simulink model "nominal_drift_REALTIME"  (R2020b)
settings: Solver=FixedStepDiscrete  StartTime=0.0  StopTime=10.0  RelTol=1e-3  EnableMultiTasking=on
values from neighbouring files (symbols this model uses):
  denHw = [0.03 0 0 0]    [data_v2_500.mat]    (also in data_v6_nominaldrift500.mat)
  denLPFz = [1 -0.978482055734]    [data_v2_500.mat]    (also in data_v6_nominaldrift500.mat)
  drv =     [data_v2_500.mat]    (also in data_v6_nominaldrift500.mat)
  gbox =     [data_v2_500.mat]    (also in data_v6_nominaldrift500.mat)
  N_u = 0    [data_v2_500.mat]    (also in data_v6_nominaldrift500.mat)
  N_x = [1 0 0 0]    [data_v2_500.mat]    (also in data_v6_nominaldrift500.mat)
  numHw = [1 0 0 -1]    [data_v2_500.mat]    (also in data_v6_nominaldrift500.mat)
  numLPFz = [0.0215179442657 0]    [data_v2_500.mat]    (also in data_v6_nominaldrift500.mat)
  sens =     [data_v2_500.mat]    (also in data_v6_nominaldrift500.mat)
  Ts = 0.01    [data_v2_500.mat]    (also in data_v6_nominaldrift500.mat)
  wheel =     [data_v2_500.mat]    (also in data_v6_nominaldrift500.mat)
undefined symbols (not defined in the file or in its folder): C_gain, DiscIntNeverNeededParam, T
libraries: BalRobTbx_baselib x9
settings Model: SILPILModeSetting=veronly  ExtModeTrigDuration=2  Creator=39345  LastModifiedBy=pavarinlau
settings DataIOCC: ReturnWorkspaceOutputs=off
settings OptimizationCC: EnhancedBackFolding=on  PassReuseOutputArgsAs=Individual arguments  ZeroExternalMemoryAtStartup=off  ZeroInternalMemoryAtStartup=off  MaxStackSize=64  OptimizeBlockOrder=speed  DifferentSizesBufferReuse=on  OptimizationCustomize=off  EfficientTunableParamExpr=on
settings DebuggingCC: ParameterTunabilityLossMsg=error
settings HardwareCC: ProdBitPerInt=16  ProdBitPerPointer=16  ProdBitPerSizeT=16  ProdBitPerPtrDiffT=16  ProdLargestAtomicFloat=None  ProdWordSize=8  ProdHWDeviceType=Atmel->AVR
settings SFSimCC: MATLABDynamicMemAlloc=off
settings RTWCC: Description=Embedded Coder  SystemTargetFile=ert.tlc  HardwareBoard=Arduino Mega 2560  TemplateMakefile=ert_default_tmf  GenerateReport=on  Toolchain=Arduino AVR  BuildConfiguration=Faster Runs
settings CodeAppCC: ForceParamTrailComments=on  IgnoreCustomStorageClasses=off  OperatorAnnotations=on  SimulinkDataObjDesc=on  SFDataObjDesc=on  InsertBlockDesc=on
settings ERTTargetCC: SupportContinuousTime=on  SupportVariableSizeSignals=on  ExtModeStaticAllocSize=2048

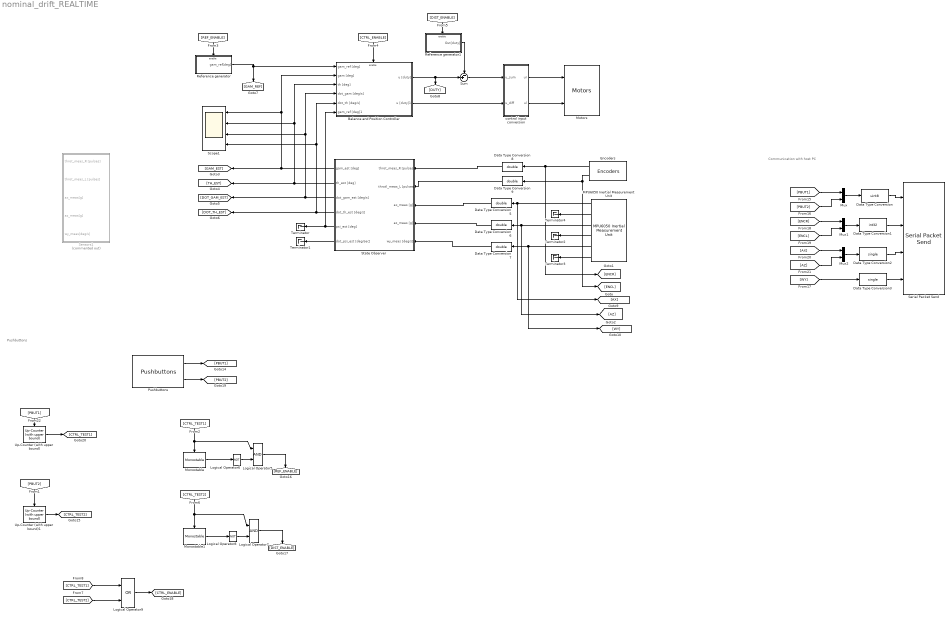
== system nominal_drift_REALTIME ==
  note: Communication with host PC
  note: Pushbuttons
  Balance and Position Controller : Subsystem
  Data Type Conversion : DataTypeConversion  OutDataTypeStr=uint8
  Data Type Conversion1 : DataTypeConversion  OutDataTypeStr=int32
  Data Type Conversion2 : DataTypeConversion  OutDataTypeStr=single
  Data Type Conversion3 : DataTypeConversion  OutDataTypeStr=single
  Data Type Conversion{5..9} (5 alike) : DataTypeConversion  OutDataTypeStr=double
  Encoders : BalRobTbx_baselib/Inputs/Encoders
      settings: SourceProductName=Balancing Robot Toolbox
  Logical Operator5 : Logic  AllPortsSameDT=off  OutDataTypeStr=boolean
  Logical Operator6 : Logic  Operator=NOT  Inputs=1  AllPortsSameDT=off  OutDataTypeStr=boolean
  Logical Operator7 : Logic  AllPortsSameDT=off  OutDataTypeStr=boolean
  Logical Operator8 : Logic  Operator=NOT  Inputs=1  AllPortsSameDT=off  OutDataTypeStr=boolean
  Logical Operator9 : Logic  Operator=OR  AllPortsSameDT=off  OutDataTypeStr=boolean
  MPU6050 Inertial Measurement Unit : BalRobTbx_baselib/Inputs/MPU6050 Inertial Measurement Unit
      settings: SourceProductName=Balancing Robot Toolbox
  Monostable : BalRobTbx_baselib/Utilities/Monostable  Tp=10
      settings: SourceProductName=Balancing Robot Toolbox
  Monostable1 : BalRobTbx_baselib/Utilities/Monostable  Tp=10
      settings: SourceProductName=Balancing Robot Toolbox
  Motors : BalRobTbx_baselib/Outputs/Motors
      settings: SourceProductName=Balancing Robot Toolbox
  Mux : Mux  Inputs=2
  Mux1 : Mux  Inputs=2
  Mux2 : Mux  Inputs=2
  Pushbuttons : BalRobTbx_baselib/Inputs/Pushbuttons
      settings: SourceProductName=Balancing Robot Toolbox
  Reference generator : Subsystem
  Reference generator1 : Subsystem
  Scope1 : Scope  NumInputPorts=4
  Sensors1 : Subsystem  Commented=on
  Serial Packet Send : BalRobTbx_baselib/Communication/Serial Packet Send  serialLinkOpt=Bluetooth  baudRateOpt=38400  waitHostTxCmd=on  txStartCmd=65  txStopCmd=66  packetSpec={'2*uint8', '2*int32', '2*single', 'single'}  cobsEncoded=on  nullTerminated=on  showEnablePort=off
      settings: SourceProductName=Balancing Robot Toolbox
  State Observer : Subsystem
  Sum : Sum  Inputs=-+|
  Terminator{,1..4} (5 alike) : Terminator
  Up-Counter (with upper bound) : BalRobTbx_baselib/Utilities/Up-Counter (with upper bound)  CMAX=10  C0=0
      settings: SourceProductName=Balancing Robot Toolbox
  Up-Counter (with upper bound)1 : BalRobTbx_baselib/Utilities/Up-Counter (with upper bound)  CMAX=10  C0=0
      settings: SourceProductName=Balancing Robot Toolbox
  control input conversion : Subsystem
  wires:
  Balance and Position Controller/2(u [duty]1) -> control input conversion/2(u_diff)
  State Observer/5(psi_est [deg]) -> Terminator/1, Balance and Position Controller/6(gam_ref [deg]1)
  [REF_ENABLE] -> Reference generator/Enable
  State Observer/1(gam_est [deg]) -> Balance and Position Controller/2(gam [deg]), Scope1/1, [GAM_EST]
  State Observer/2(th_est [deg]) -> Balance and Position Controller/3(th [deg]), Scope1/2, [TH_EST]
  Data Type Conversion6/1 -> State Observer/4("az_meas [g] ")
  Reference generator/1(gam_ref[deg]) -> Balance and Position Controller/1(gam_ref [deg]), [GAM_REF]
  [CTRL_ENABLE] -> Balance and Position Controller/Enable
  Sum/1 -> control input conversion/1(u_sum)
  Data Type Conversion9/1 -> State Observer/2(throtl_meas_L [pulses])
  State Observer/4(dot_th_est [deg/s]) -> Balance and Position Controller/5(dot_th [deg/s]), Scope1/4, [DOT_TH_EST]
  Reference generator1/1(Out[duty]) -> Sum/1
  State Observer/6(dot_psi_est [deg/sec]) -> Terminator1/1
  Data Type Conversion8/1 -> State Observer/1("throt_meas_R [pulses] ")
  State Observer/3(dot_gam_est [deg/s]) -> Balance and Position Controller/4(dot_gam [deg/s]), Scope1/3, [DOT_GAM_EST]
  Data Type Conversion7/1 -> State Observer/5(wy_meas [deg/s])
  [DIST_ENABLE] -> Reference generator1/Enable
  Balance and Position Controller/1(u [duty]) -> [DUTY], Sum/2
  Data Type Conversion3/1 -> Serial Packet Send/4
  Mux2/1 -> Data Type Conversion2/1
  Data Type Conversion2/1 -> Serial Packet Send/3
  [WY] -> Data Type Conversion3/1
  Data Type Conversion1/1 -> Serial Packet Send/2
  [ENCR] -> Mux1/1
  [PBUT2] -> Mux/2
  [PBUT1] -> Mux/1
  Mux/1 -> Data Type Conversion/1
  [AX] -> Mux2/1
  [ENCL] -> Mux1/2
  [AZ] -> Mux2/2
  Data Type Conversion/1 -> Serial Packet Send/1
  Mux1/1 -> Data Type Conversion1/1
  [PBUT1] -> Up-Counter (with upper bound)/Trigger
  Up-Counter (with upper bound)/1 -> [CTRL_TEST1]
  Up-Counter (with upper bound)1/1 -> [CTRL_TEST2]
  Monostable/1 -> Logical Operator6/1
  Pushbuttons/2 -> [PBUT2]
  Logical Operator7/1 -> [DIST_ENABLE]
  Pushbuttons/1 -> [PBUT1]
  [CTRL_TEST2] -> Logical Operator9/2
  Logical Operator6/1 -> Logical Operator5/2
  [CTRL_TEST2] -> Logical Operator7/1, Monostable1/Enable
  Logical Operator9/1 -> [CTRL_ENABLE]
  [PBUT2] -> Up-Counter (with upper bound)1/Trigger
  [CTRL_TEST1] -> Monostable/Enable, Logical Operator5/1
  [CTRL_TEST1] -> Logical Operator9/1
  Logical Operator5/1 -> [REF_ENABLE]
  Monostable1/1 -> Logical Operator8/1
  Logical Operator8/1 -> Logical Operator7/2
  Encoders/1 -> [ENCR], Data Type Conversion8/1
  MPU6050 Inertial Measurement Unit/5 -> [WY], Data Type Conversion7/1
  MPU6050 Inertial Measurement Unit/2 -> Terminator4/1
  MPU6050 Inertial Measurement Unit/3 -> [AZ], Data Type Conversion6/1
  MPU6050 Inertial Measurement Unit/6 -> Terminator3/1
  MPU6050 Inertial Measurement Unit/1 -> [AX], Data Type Conversion5/1
  MPU6050 Inertial Measurement Unit/4 -> Terminator2/1
  Encoders/2 -> [ENCL], Data Type Conversion9/1
  Data Type Conversion5/1 -> State Observer/3("ax_meas [g] ")
  control input conversion/1(ur) -> Motors/1
  control input conversion/2(ul) -> Motors/2

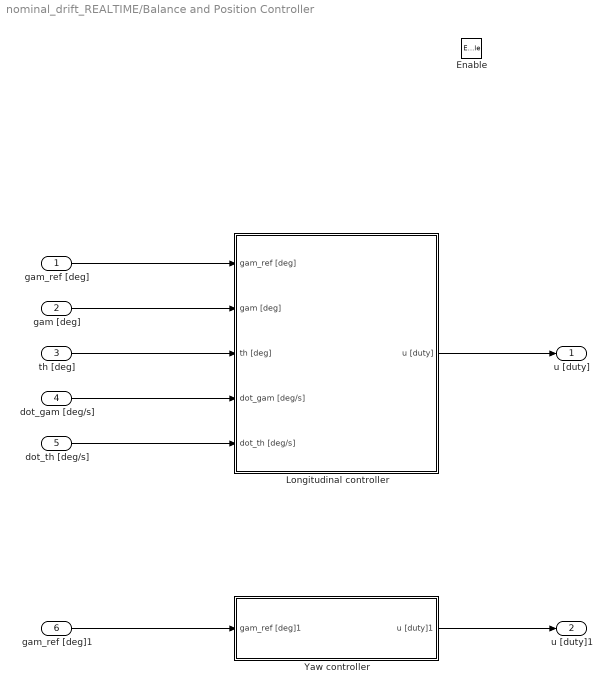
== system nominal_drift_REALTIME/Balance and Position Controller ==
  gam_ref [deg] : Inport
  gam [deg] : Inport  Port=2
  th [deg] : Inport  Port=3
  dot_gam [deg/s] : Inport  Port=4
  dot_th [deg/s] : Inport  Port=5
  gam_ref [deg]1 : Inport  Port=6
  Enable : EnablePort  StatesWhenEnabling=reset
  Longitudinal controller : Subsystem
  Yaw controller : Subsystem
  u [duty] : Outport
  u [duty]1 : Outport  Port=2  InitialOutput=[0]
  wires:
  gam_ref [deg]/1 -> Longitudinal controller/1(gam_ref [deg])
  Longitudinal controller/1(u [duty]) -> u [duty]/1
  gam [deg]/1 -> Longitudinal controller/2(gam [deg])
  th [deg]/1 -> Longitudinal controller/3(th [deg])
  dot_th [deg/s]/1 -> Longitudinal controller/5(dot_th [deg/s])
  dot_gam [deg/s]/1 -> Longitudinal controller/4(dot_gam [deg/s])
  Yaw controller/1(u [duty]1) -> u [duty]1/1
  gam_ref [deg]1/1 -> Yaw controller/1(gam_ref [deg]1)

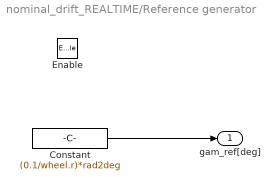
== system nominal_drift_REALTIME/Reference generator ==
  Enable : EnablePort  StatesWhenEnabling=reset
  Constant : Constant  Value=(0.1/wheel.r)*rad2deg  SampleTime=0.01
  gam_ref[deg] : Outport
  wires:
  Constant/1 -> gam_ref[deg]/1

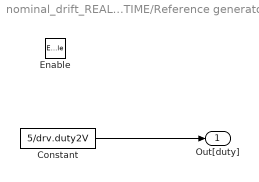
== system nominal_drift_REALTIME/Reference generator1 ==
  Enable : EnablePort  StatesWhenEnabling=reset
  Constant : Constant  Value=5/drv.duty2V  SampleTime=0.01
  Out[duty] : Outport  InitialOutput=[0]
  wires:
  Constant/1 -> Out[duty]/1

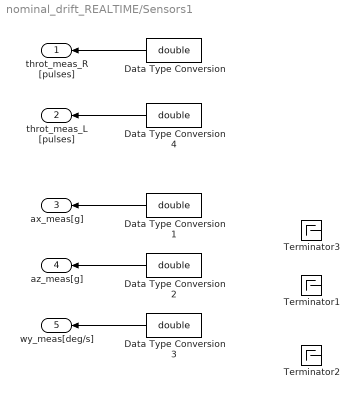
== system nominal_drift_REALTIME/Sensors1 ==
  Data Type Conversion{,1..4} (5 alike) : DataTypeConversion  OutDataTypeStr=double
  Terminator1 : Terminator
  Terminator2 : Terminator
  Terminator3 : Terminator
  throt_meas_R [pulses] : Outport
  throt_meas_L [pulses] : Outport  Port=2
  ax_meas[g] : Outport  Port=3
  az_meas[g] : Outport  Port=4
  wy_meas[deg/s] : Outport  Port=5
  wires:
  Data Type Conversion/1 -> throt_meas_R [pulses]/1
  Data Type Conversion1/1 -> ax_meas[g]/1
  Data Type Conversion2/1 -> az_meas[g]/1
  Data Type Conversion3/1 -> wy_meas[deg/s]/1
  Data Type Conversion4/1 -> throt_meas_L [pulses]/1

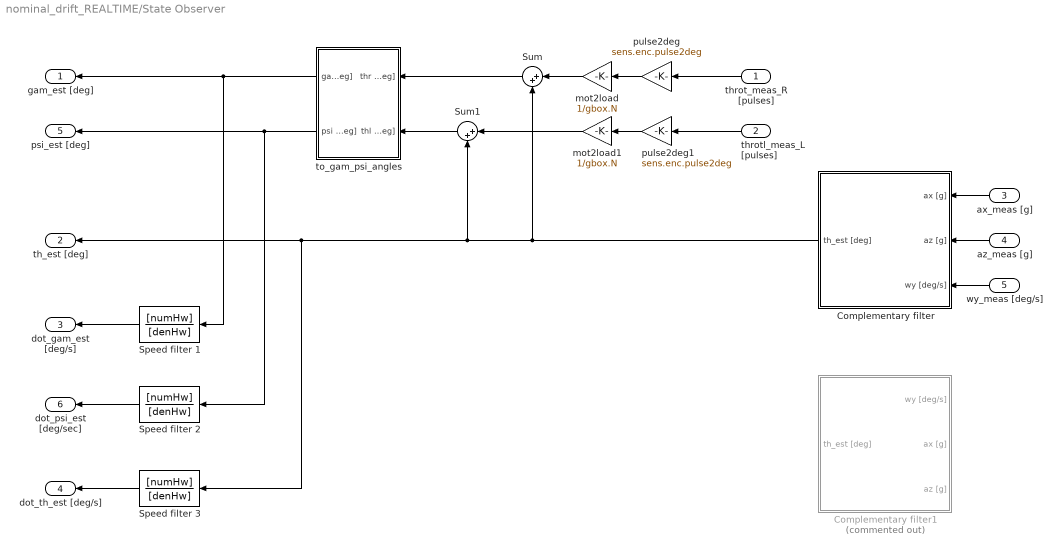
== system nominal_drift_REALTIME/State Observer ==
  "throt_meas_R [pulses] " : Inport
  throtl_meas_L [pulses] : Inport  Port=2
  "ax_meas [g] " : Inport  Port=3
  "az_meas [g] " : Inport  Port=4
  wy_meas [deg/s] : Inport  Port=5
  Complementary filter : Subsystem
  Complementary filter1 : Subsystem  Commented=on
  Speed filter 1 : DiscreteTransferFcn  Numerator=[numHw]  Denominator=[denHw]  SampleTime=Ts
  Speed filter 2 : DiscreteTransferFcn  Numerator=[numHw]  Denominator=[denHw]  SampleTime=Ts
  Speed filter 3 : DiscreteTransferFcn  Numerator=[numHw]  Denominator=[denHw]  SampleTime=Ts
  Sum : Sum  Inputs=|++
  Sum1 : Sum  Inputs=|++
  mot2load : Gain  Gain=1/gbox.N
  mot2load1 : Gain  Gain=1/gbox.N
  pulse2deg : Gain  Gain=sens.enc.pulse2deg
  pulse2deg1 : Gain  Gain=sens.enc.pulse2deg
  to_gam_psi_angles : Subsystem
  gam_est [deg] : Outport
  th_est [deg] : Outport  Port=2
  dot_gam_est [deg/s] : Outport  Port=3
  dot_th_est [deg/s] : Outport  Port=4
  psi_est [deg] : Outport  Port=5
  dot_psi_est [deg/sec] : Outport  Port=6
  wires:
  pulse2deg/1 -> mot2load/1
  "throt_meas_R [pulses] "/1 -> pulse2deg/1
  mot2load/1 -> Sum/1
  Complementary filter/1("th_est [deg] ") -> Sum/2, th_est [deg]/1, Speed filter 3/1, Sum1/2
  Speed filter 1/1 -> dot_gam_est [deg/s]/1
  Speed filter 3/1 -> dot_th_est [deg/s]/1
  "ax_meas [g] "/1 -> Complementary filter/1("ax [g] ")
  "az_meas [g] "/1 -> Complementary filter/2("az [g] ")
  wy_meas [deg/s]/1 -> Complementary filter/3(wy [deg/s])
  throtl_meas_L [pulses]/1 -> pulse2deg1/1
  pulse2deg1/1 -> mot2load1/1
  mot2load1/1 -> Sum1/1
  Sum1/1 -> to_gam_psi_angles/2(thl [deg])
  Sum/1 -> to_gam_psi_angles/1(thr [deg])
  to_gam_psi_angles/1(gam [deg]) -> Speed filter 1/1, gam_est [deg]/1
  to_gam_psi_angles/2(psi [deg]) -> Speed filter 2/1, psi_est [deg]/1
  Speed filter 2/1 -> dot_psi_est [deg/sec]/1

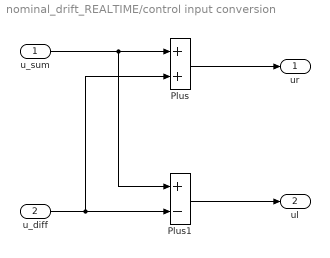
== system nominal_drift_REALTIME/control input conversion ==
  u_sum : Inport
  u_diff : Inport  Port=2
  Plus : Sum
  Plus1 : Sum  Inputs=+-
  ur : Outport
  ul : Outport  Port=2
  wires:
  u_sum/1 -> Plus1/1, Plus/1
  u_diff/1 -> Plus1/2, Plus/2
  Plus/1 -> ur/1
  Plus1/1 -> ul/1

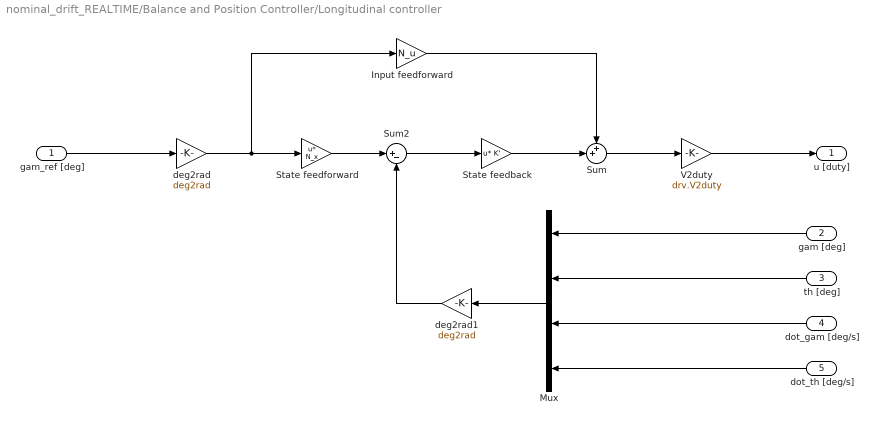
== system nominal_drift_REALTIME/Balance and Position Controller/Longitudinal controller ==
  gam_ref [deg] : Inport
  gam [deg] : Inport  Port=2
  th [deg] : Inport  Port=3
  dot_gam [deg/s] : Inport  Port=4
  dot_th [deg/s] : Inport  Port=5
  Input feedforward : Gain  Gain=N_u
  Mux : Mux
  State feedback : Gain  Gain=K'  Multiplication=Matrix(u*K)
  "State feedforward\t" : Gain  Gain=N_x  Multiplication=Matrix(u*K)
  Sum : Sum  Inputs=++|
  Sum2 : Sum  Inputs=|+-
  V2duty : Gain  Gain=drv.V2duty
  deg2rad : Gain  Gain=deg2rad
  deg2rad1 : Gain  Gain=deg2rad
  u [duty] : Outport
  wires:
  Mux/1 -> deg2rad1/1
  Sum2/1 -> State feedback/1
  deg2rad/1 -> Input feedforward/1, "State feedforward\t"/1
  dot_gam [deg/s]/1 -> Mux/3
  State feedback/1 -> Sum/2
  "State feedforward\t"/1 -> Sum2/1
  deg2rad1/1 -> Sum2/2
  Sum/1 -> V2duty/1
  dot_th [deg/s]/1 -> Mux/4
  Input feedforward/1 -> Sum/1
  gam_ref [deg]/1 -> deg2rad/1
  gam [deg]/1 -> Mux/1
  th [deg]/1 -> Mux/2
  V2duty/1 -> u [duty]/1

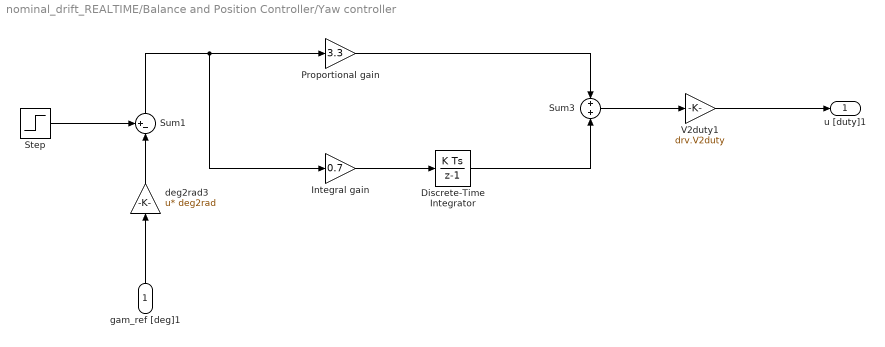
== system nominal_drift_REALTIME/Balance and Position Controller/Yaw controller ==
  gam_ref [deg]1 : Inport
  Discrete-Time Integrator : DiscreteIntegrator  SampleTime=-1  ICPrevOutput=DiscIntNeverNeededParam  ICPrevScaledInput=DiscIntNeverNeededParam
  Integral gain : Gain  Gain=0.7
  Proportional gain : Gain  Gain=3.3
  Step : Step  Time=0  After=0  SampleTime=0
  Sum1 : Sum  Inputs=+-|
  Sum3 : Sum  Inputs=+|+
  V2duty1 : Gain  Gain=drv.V2duty
  deg2rad3 : Gain  Gain=deg2rad  Multiplication=Matrix(u*K)
  u [duty]1 : Outport
  wires:
  gam_ref [deg]1/1 -> deg2rad3/1
  Sum1/1 -> Integral gain/1, Proportional gain/1
  Step/1 -> Sum1/1
  Integral gain/1 -> Discrete-Time Integrator/1
  deg2rad3/1 -> Sum1/2
  V2duty1/1 -> u [duty]1/1
  Proportional gain/1 -> Sum3/1
  Discrete-Time Integrator/1 -> Sum3/2
  Sum3/1 -> V2duty1/1

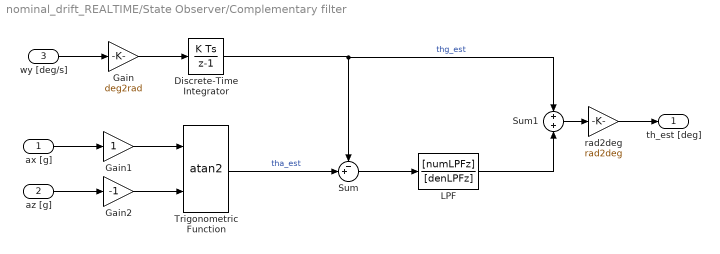
== system nominal_drift_REALTIME/State Observer/Complementary filter ==
  "ax [g] " : Inport
  "az [g] " : Inport  Port=2
  wy [deg/s] : Inport  Port=3
  Discrete-Time Integrator : DiscreteIntegrator  gainval=1  SampleTime=Ts  ICPrevOutput=DiscIntNeverNeededParam  ICPrevScaledInput=DiscIntNeverNeededParam
  Gain : Gain  Gain=deg2rad
  Gain1 : Gain
  Gain2 : Gain  Gain=-1
  LPF : DiscreteTransferFcn  Numerator=[numLPFz]  Denominator=[denLPFz]  SampleTime=Ts
  Sum : Sum  Inputs=-+|
  Sum1 : Sum
  Trigonometric Function : Trigonometry  Operator=atan2
  rad2deg : Gain  Gain=rad2deg
  "th_est [deg] " : Outport
  wires:
  "az [g] "/1 -> Gain2/1
  "ax [g] "/1 -> Gain1/1
  wy [deg/s]/1 -> Gain/1
  Gain/1 -> Discrete-Time Integrator/1
  Gain2/1 -> Trigonometric Function/2
  Gain1/1 -> Trigonometric Function/1
  Trigonometric Function/1 -> Sum/2  "tha_est"
  Discrete-Time Integrator/1 -> Sum1/1, Sum/1  "thg_est"
  rad2deg/1 -> "th_est [deg] "/1
  Sum1/1 -> rad2deg/1
  Sum/1 -> LPF/1
  LPF/1 -> Sum1/2

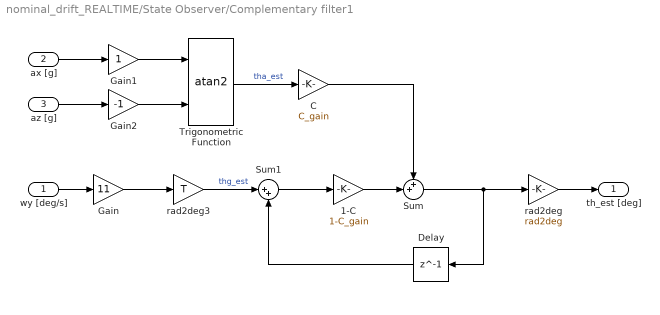
== system nominal_drift_REALTIME/State Observer/Complementary filter1 ==
  wy [deg/s] : Inport
  "ax [g] " : Inport  Port=2
  "az [g] " : Inport  Port=3
  1-C : Gain  Gain=1-C_gain
  C : Gain  Gain=C_gain
  Delay : Delay  DelayLength=1
  Gain : Gain  Gain=11
  Gain1 : Gain
  Gain2 : Gain  Gain=-1
  Sum : Sum  Inputs=++|
  Sum1 : Sum  Inputs=|++
  Trigonometric Function : Trigonometry  Operator=atan2
  rad2deg : Gain  Gain=rad2deg
  rad2deg3 : Gain  Gain=T
  "th_est [deg] " : Outport
  wires:
  "az [g] "/1 -> Gain2/1
  "ax [g] "/1 -> Gain1/1
  wy [deg/s]/1 -> Gain/1
  Gain/1 -> rad2deg3/1
  Gain2/1 -> Trigonometric Function/2
  Gain1/1 -> Trigonometric Function/1
  rad2deg/1 -> "th_est [deg] "/1
  Trigonometric Function/1 -> C/1  "tha_est"
  C/1 -> Sum/1
  1-C/1 -> Sum/2
  Sum/1 -> Delay/1, rad2deg/1
  Delay/1 -> Sum1/2
  rad2deg3/1 -> Sum1/1  "thg_est"
  Sum1/1 -> 1-C/1

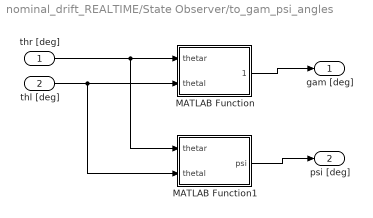
== system nominal_drift_REALTIME/State Observer/to_gam_psi_angles ==
  thr [deg] : Inport
  thl [deg] : Inport  Port=2
  MATLAB Function : MATLAB Function  TreatAsAtomicUnit=on
  MATLAB Function1 : MATLAB Function  TreatAsAtomicUnit=on
  gam [deg] : Outport
  psi [deg] : Outport  Port=2
  wires:
  thr [deg]/1 -> MATLAB Function1/1(thetar), MATLAB Function/1(thetar)
  thl [deg]/1 -> MATLAB Function1/2(thetal), MATLAB Function/2(thetal)
  MATLAB Function/1(gamma) -> gam [deg]/1
  MATLAB Function1/1(psi) -> psi [deg]/1

== matlab function nominal_drift_REALTIME/State Observer/to_gam_psi_angles/MATLAB Function ==
  data: thetar input; gamma output; thetal input
function gamma = fcn(thetar, thetal)
gamma = (thetar+thetal)/2;

== matlab function nominal_drift_REALTIME/State Observer/to_gam_psi_angles/MATLAB Function1 ==
  data: thetar input; thetal input; psi output
function psi = fcn(thetar, thetal)
diff = thetar - thetal;
psi = 34e-3*diff/(100e-3*2);
